simulink model "triplex_12B"  (R2024b)
settings: Solver=ode3  StartTime=0.0  StopTime=10.0  FixedStep=.1  RelTol=1e-3  EnableMultiTasking=on
settings Model: Creator=elliocm  LastModifiedBy=lukeubun
settings SolverCC: AlgebraicLoopSolver=TrustRegion
settings DataIOCC: LimitDataPoints=on  SaveFormat=StructureWithTime  SignalLoggingSaveFormat=ModelDataLogs  ReturnWorkspaceOutputs=off
settings OptimizationCC: ExpressionDepthLimit=2147483647  LifeSpan=inf
settings DebuggingCC: UnderspecifiedInitializationDetection=Classic  MergeDetectMultiDrivingBlocksExec=none  SolverPrmCheckMsg=warning  MultiTaskDSMMsg=warning  MultiTaskCondExecSysMsg=none  UnconnectedInputMsg=warning  UnconnectedOutputMsg=warning  UnconnectedLineMsg=warning  StateNameClashWarn=warning  SFUnexpectedBacktrackingDiag=warning  SFNoUnconditionalDefaultTransitionDiag=warning  SFExecutionAtInitializationDiag=none  ArithmeticOperatorsInVariantConditions=warning
settings HardwareCC: ProdBitPerPointer=32  ProdBitPerSizeT=32  ProdBitPerPtrDiffT=32  ProdLargestAtomicFloat=None  ProdIntDivRoundTo=Undefined  ProdEndianess=Unspecified  ProdWordSize=32  ProdHWDeviceType=32-bit Generic
settings ModelReferenceCC: PropagateSignalLabelsOutOfModel=off
settings SFSimCC: SimUseLocalCustomCode=off  CustomCodeUndefinedFunction=UseInterfaceOnly
settings RTWCC: RTWUseLocalCustomCode=off  GPUComputeCapability=3.5
settings CodeAppCC: StateflowObjectComments=on
settings GRTTargetCC: TargetLangStandard=C89/C90 (ANSI)
settings ConfigComp: CovMetricSettings=dw  CovSaveCumulativeToWorkspaceVar=on  CovSaveSingleToWorkspaceVar=on  CovExternalEMLEnable=off

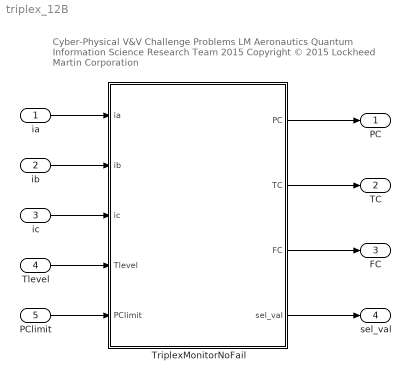
== system triplex_12B ==
  note: Cyber-Physical V&V Challenge Problems
      | LM Aeronautics Quantum Information Science Research Team 2015
      | Copyright © 2015 Lockheed Martin Corporation
  ia : Inport  OutDataTypeStr=double
  ib : Inport  Port=2  OutDataTypeStr=double
  ic : Inport  Port=3  OutDataTypeStr=double
  Tlevel : Inport  Port=4  OutDataTypeStr=double
  PClimit : Inport  Port=5  OutDataTypeStr=int32
  TriplexMonitorNoFail : Subsystem
  PC : Outport
  TC : Outport  Port=2
  FC : Outport  Port=3
  sel_val : Outport  Port=4
  wires:
  ia/1 -> TriplexMonitorNoFail/1(ia)
  ib/1 -> TriplexMonitorNoFail/2(ib)
  ic/1 -> TriplexMonitorNoFail/3(ic)
  Tlevel/1 -> TriplexMonitorNoFail/4(Tlevel)
  PClimit/1 -> TriplexMonitorNoFail/5(PClimit)
  TriplexMonitorNoFail/2(TC) -> TC/1
  TriplexMonitorNoFail/1(PC) -> PC/1
  TriplexMonitorNoFail/3(FC) -> FC/1
  TriplexMonitorNoFail/4(sel_val) -> sel_val/1

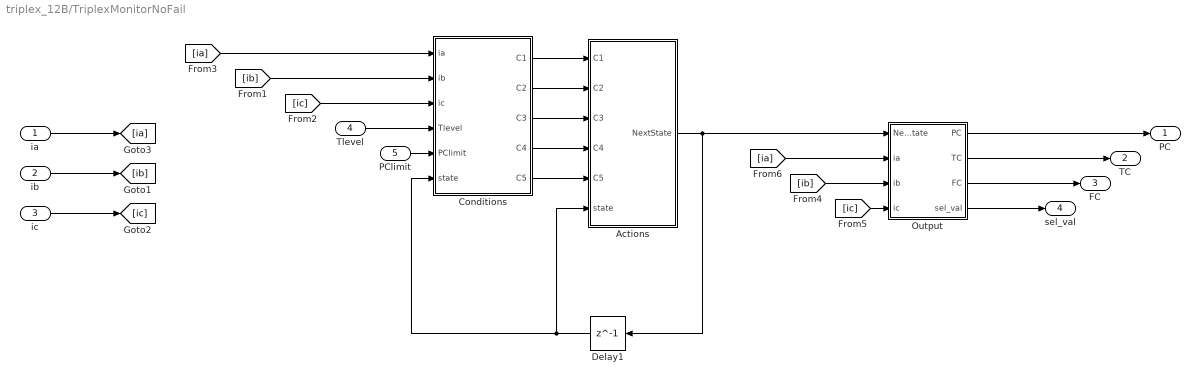
== system triplex_12B/TriplexMonitorNoFail ==
  ia : Inport
  ib : Inport  Port=2
  ic : Inport  Port=3
  Tlevel : Inport  Port=4
  PClimit : Inport  Port=5
  Actions : Subsystem
  Conditions : Subsystem
  Delay1 : Delay  DelayLength=1  InitialCondition=0
  Output : Subsystem
  PC : Outport
  TC : Outport  Port=2
  FC : Outport  Port=3
  sel_val : Outport  Port=4
  wires:
  Conditions/2(C2) -> Actions/2(C2)
  Conditions/5(C5) -> Actions/5(C5)
  Conditions/1(C1) -> Actions/1(C1)
  Conditions/4(C4) -> Actions/4(C4)
  Conditions/3(C3) -> Actions/3(C3)
  Tlevel/1 -> Conditions/4(Tlevel)
  PClimit/1 -> Conditions/5(PClimit)
  Output/2(TC) -> TC/1
  Output/1(PC) -> PC/1
  Output/3(FC) -> FC/1
  Actions/1(NextState) -> Delay1/1, Output/1(NextState)
  Delay1/1 -> Actions/6(state), Conditions/6(state)
  [ia] -> Conditions/1(ia)
  [ib] -> Conditions/2(ib)
  ib/1 -> [ib]
  ic/1 -> [ic]
  [ic] -> Conditions/3(ic)
  [ia] -> Output/2(ia)
  [ib] -> Output/3(ib)
  [ic] -> Output/4(ic)
  Output/4(sel_val) -> sel_val/1
  ia/1 -> [ia]

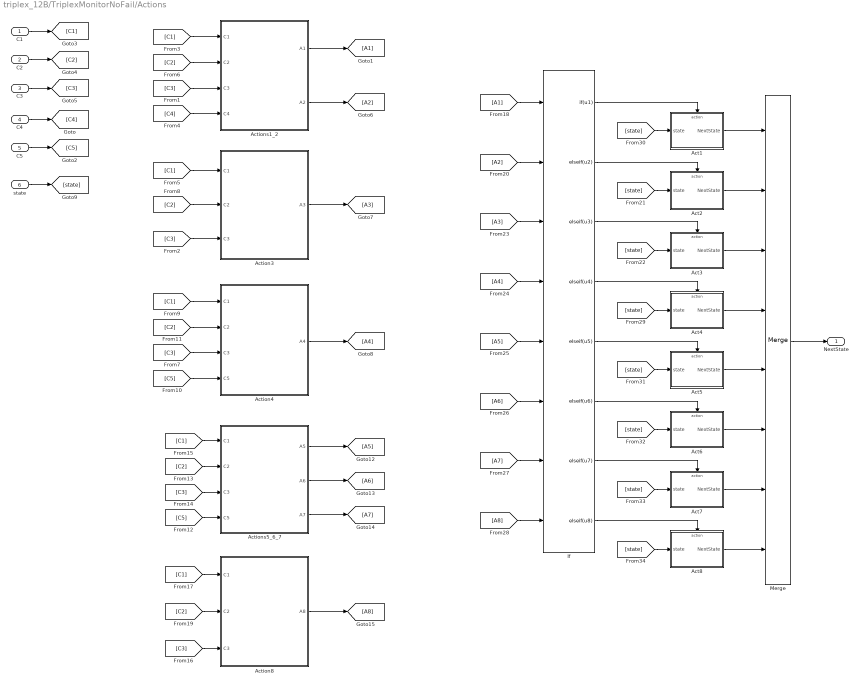
== system triplex_12B/TriplexMonitorNoFail/Actions ==
  C1 : Inport
  C2 : Inport  Port=2
  C3 : Inport  Port=3
  C4 : Inport  Port=4
  C5 : Inport  Port=5
  state : Inport  Port=6
  Act1 : Subsystem
  Act2 : Subsystem
  Act3 : Subsystem
  Act4 : Subsystem
  Act5 : Subsystem
  Act6 : Subsystem
  Act7 : Subsystem
  Act8 : Subsystem
  Action3 : Subsystem
  Action4 : Subsystem
  Action8 : Subsystem
  Actions1_2 : Subsystem
  Actions5_6_7 : Subsystem
  If : If  NumInputs=8  IfExpression=u1  ElseIfExpressions=u2, u3, u4, u5, u6, u7, u8  ShowElse=off
  Merge : Merge  Inputs=8
  NextState : Outport
  wires:
  C1/1 -> [C1]
  C5/1 -> [C5]
  C2/1 -> [C2]
  C3/1 -> [C3]
  C4/1 -> [C4]
  [C1] -> Actions1_2/1(C1)
  [C2] -> Actions1_2/2(C2)
  [C4] -> Actions1_2/4(C4)
  [C3] -> Actions1_2/3(C3)
  Actions1_2/2(A2) -> [A2]
  [C1] -> Action3/1(C1)
  [C2] -> Action3/2(C2)
  [C3] -> Action3/3(C3)
  Action4/1(A4) -> [A4]
  [C1] -> Action4/1(C1)
  [C2] -> Action4/2(C2)
  [C3] -> Action4/3(C3)
  [C5] -> Action4/4(C5)
  [C2] -> Actions5_6_7/2(C2)
  [C3] -> Actions5_6_7/3(C3)
  [C1] -> Actions5_6_7/1(C1)
  [C5] -> Actions5_6_7/4(C5)
  [C1] -> Action8/1(C1)
  [C2] -> Action8/2(C2)
  [C3] -> Action8/3(C3)
  Actions1_2/1(A1) -> [A1]
  Action3/1(A3) -> [A3]
  [A1] -> If/1
  If/1 -> Act1/Action
  [A2] -> If/2
  state/1 -> [state]
  If/2 -> Act2/Action
  If/3 -> Act3/Action
  [A3] -> If/3
  [A4] -> If/4
  [A5] -> If/5
  [A6] -> If/6
  [A7] -> If/7
  [A8] -> If/8
  If/4 -> Act4/Action
  Actions5_6_7/1(A5) -> [A5]
  Actions5_6_7/2(A6) -> [A6]
  Actions5_6_7/3(A7) -> [A7]
  Action8/1(A8) -> [A8]
  [state] -> Act1/1(state)
  If/5 -> Act5/Action
  If/6 -> Act6/Action
  If/7 -> Act7/Action
  If/8 -> Act8/Action
  Act1/1(NextState) -> Merge/1
  Act2/1(NextState) -> Merge/2
  Act3/1(NextState) -> Merge/3
  Act4/1(NextState) -> Merge/4
  Act5/1(NextState) -> Merge/5
  Act6/1(NextState) -> Merge/6
  Act7/1(NextState) -> Merge/7
  Act8/1(NextState) -> Merge/8
  Merge/1 -> NextState/1
  [state] -> Act2/1(state)
  [state] -> Act3/1(state)
  [state] -> Act4/1(state)
  [state] -> Act5/1(state)
  [state] -> Act6/1(state)
  [state] -> Act7/1(state)
  [state] -> Act8/1(state)

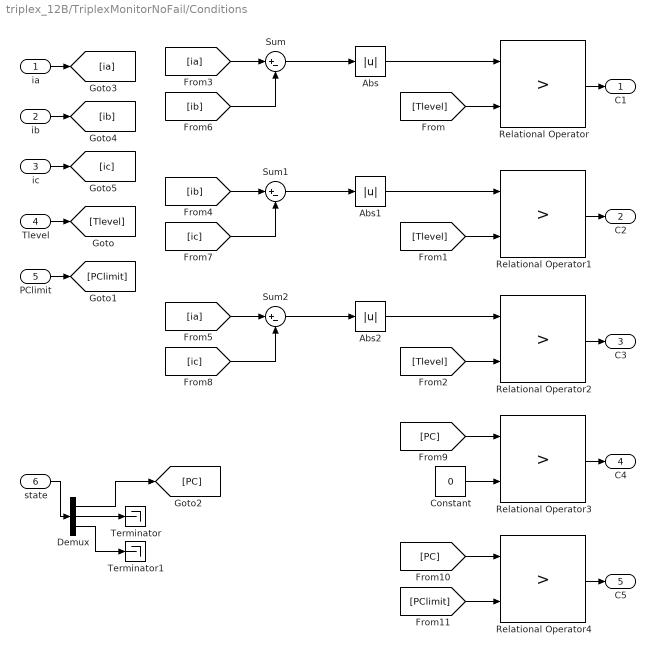
== system triplex_12B/TriplexMonitorNoFail/Conditions ==
  ia : Inport  Tag=ia
  ib : Inport  Port=2
  ic : Inport  Port=3
  Tlevel : Inport  Port=4
  PClimit : Inport  Port=5
  state : Inport  Port=6
  Abs : Abs  SaturateOnIntegerOverflow=off
  Abs1 : Abs  SaturateOnIntegerOverflow=off
  Abs2 : Abs  SaturateOnIntegerOverflow=off
  Constant : Constant  Value=0
  Demux : Demux  Outputs=3
  Relational Operator{,1..4} (5 alike) : RelationalOperator  Operator=>  OutDataTypeStr=boolean  InputSameDT=off
  Sum : Sum  Inputs=|+-
  Sum1 : Sum  Inputs=|+-
  Sum2 : Sum  Inputs=|+-
  Terminator : Terminator
  Terminator1 : Terminator
  C1 : Outport
  C2 : Outport  Port=2
  C3 : Outport  Port=3
  C4 : Outport  Port=4
  C5 : Outport  Port=5
  wires:
  Abs/1 -> Relational Operator/1
  Sum/1 -> Abs/1
  [Tlevel] -> Relational Operator/2
  Constant/1 -> Relational Operator3/2
  Abs1/1 -> Relational Operator1/1
  [Tlevel] -> Relational Operator1/2
  Sum1/1 -> Abs1/1
  Sum2/1 -> Abs2/1
  Abs2/1 -> Relational Operator2/1
  [Tlevel] -> Relational Operator2/2
  Relational Operator4/1 -> C5/1
  ib/1 -> [ib]
  [ia] -> Sum/1
  Relational Operator1/1 -> C2/1
  [PC] -> Relational Operator4/1
  Tlevel/1 -> [Tlevel]
  [ic] -> Sum1/2
  ia/1 -> [ia]
  ic/1 -> [ic]
  Relational Operator2/1 -> C3/1
  [ic] -> Sum2/2
  [ia] -> Sum2/1
  [ib] -> Sum/2
  [ib] -> Sum1/1
  [PC] -> Relational Operator3/1
  Relational Operator3/1 -> C4/1
  [PClimit] -> Relational Operator4/2
  PClimit/1 -> [PClimit]
  Relational Operator/1 -> C1/1
  state/1 -> Demux/1
  Demux/1 -> [PC]
  Demux/2 -> Terminator/1
  Demux/3 -> Terminator1/1

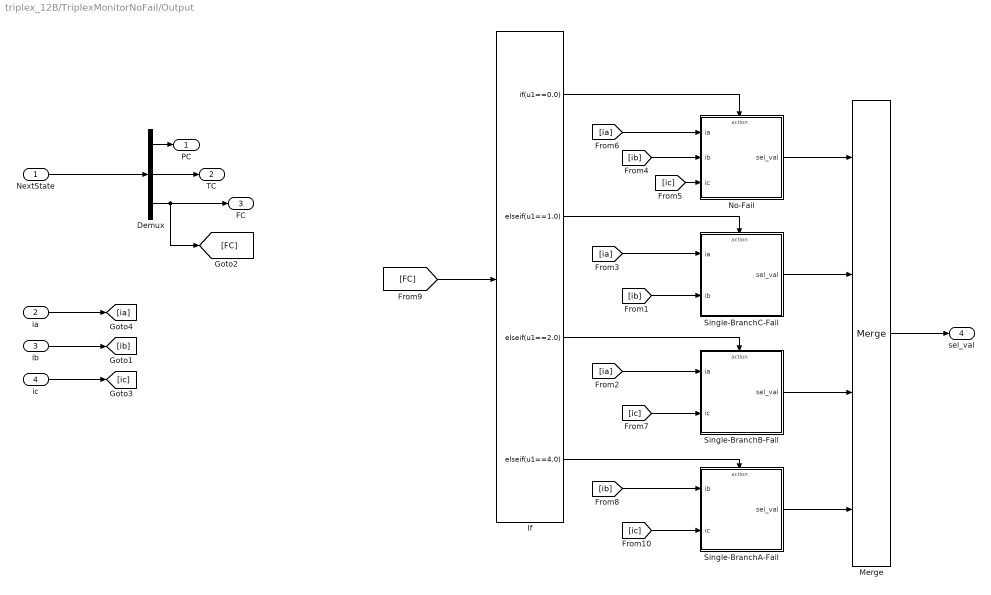
== system triplex_12B/TriplexMonitorNoFail/Output ==
  NextState : Inport
  ia : Inport  Port=2
  ib : Inport  Port=3
  ic : Inport  Port=4
  Demux : Demux  Outputs=3
  If : If  IfExpression=u1==0.0  ElseIfExpressions=u1==1.0, u1==2.0, u1==4.0  ShowElse=off
  Merge : Merge  Inputs=4
  No-Fail : Subsystem
  Single-BranchA-Fail : Subsystem
  Single-BranchB-Fail : Subsystem
  Single-BranchC-Fail : Subsystem
  PC : Outport
  TC : Outport  Port=2
  FC : Outport  Port=3
  sel_val : Outport  Port=4
  wires:
  NextState/1 -> Demux/1
  Demux/1 -> PC/1
  Demux/2 -> TC/1
  Demux/3 -> [FC], FC/1
  [FC] -> If/1
  If/1 -> No-Fail/Action
  ia/1 -> [ia]
  ib/1 -> [ib]
  ic/1 -> [ic]
  Merge/1 -> sel_val/1
  [ia] -> No-Fail/1(ia)
  [ib] -> No-Fail/2(ib)
  [ic] -> No-Fail/3(ic)
  If/2 -> Single-BranchC-Fail/Action
  [ia] -> Single-BranchC-Fail/1(ia)
  [ib] -> Single-BranchC-Fail/2(ib)
  If/3 -> Single-BranchB-Fail/Action
  [ia] -> Single-BranchB-Fail/1(ia)
  [ic] -> Single-BranchB-Fail/2(ic)
  If/4 -> Single-BranchA-Fail/Action
  [ib] -> Single-BranchA-Fail/1(ib)
  [ic] -> Single-BranchA-Fail/2(ic)
  No-Fail/1(sel_val) -> Merge/1
  Single-BranchC-Fail/1(sel_val) -> Merge/2
  Single-BranchB-Fail/1(sel_val) -> Merge/3
  Single-BranchA-Fail/1(sel_val) -> Merge/4

== system triplex_12B/TriplexMonitorNoFail/Actions/Act1 ==
  note: // Action 1: No pending failures
  state : Inport
  Action Port : ActionPort  ActionPortLabel=if(u1)
  Constant1 : Constant  Value=0  OutDataTypeStr=int32
  Demux : Demux  Outputs=3
  Mux : Mux  Inputs=3
  Signal Conversion : SignalConversion  OverrideOpt=off
  Terminator : Terminator
  NextState : Outport
  wires:
  state/1 -> [state]
  Signal Conversion/1 -> NextState/1
  Mux/1 -> Signal Conversion/1
  [state] -> Demux/1
  Demux/2 -> Mux/2
  Demux/3 -> Mux/3
  Constant1/1 -> Mux/1
  Demux/1 -> Terminator/1

== system triplex_12B/TriplexMonitorNoFail/Actions/Act2 ==
  note: // Action 2: Failure pending but no miscompares
  state : Inport
  Action Port : ActionPort  ActionPortLabel=elseif(u2)
  Constant1 : Constant  OutDataTypeStr=int32
  Demux : Demux  Outputs=3
  Mux : Mux  Inputs=3
  Signal Conversion : SignalConversion  OverrideOpt=off
  Sum : Sum  Inputs=-+|
  NextState : Outport
  wires:
  state/1 -> [state]
  Constant1/1 -> Sum/1
  Signal Conversion/1 -> NextState/1
  Mux/1 -> Signal Conversion/1
  [state] -> Demux/1
  Demux/2 -> Mux/2
  Demux/3 -> Mux/3
  Sum/1 -> Mux/1
  Demux/1 -> Sum/2

== system triplex_12B/TriplexMonitorNoFail/Actions/Act3 ==
  note: // Action 3: Do nothing there is only 1 miscompare
  state : Inport
  Action Port : ActionPort  ActionPortLabel=elseif( u3)
  NextState : Outport
  wires:
  state/1 -> NextState/1

== system triplex_12B/TriplexMonitorNoFail/Actions/Act4 ==
  note: // Action 4: Failure pending
  state : Inport
  Action Port : ActionPort  ActionPortLabel=elseif( u4)
  Constant1 : Constant  OutDataTypeStr=int32
  Demux : Demux  Outputs=3
  Mux : Mux  Inputs=3
  Signal Conversion : SignalConversion  OverrideOpt=off
  Sum : Sum  Inputs=++|
  Sum1 : Sum  Inputs=|++
  NextState : Outport
  wires:
  state/1 -> [state]
  Signal Conversion/1 -> NextState/1
  Mux/1 -> Signal Conversion/1
  [state] -> Demux/1
  Demux/2 -> Sum/2
  Constant1/1 -> Sum1/2, Sum/1
  Demux/1 -> Sum1/1
  Sum1/1 -> Mux/1
  Sum/1 -> Mux/2
  Demux/3 -> Mux/3

== system triplex_12B/TriplexMonitorNoFail/Actions/Act5 ==
  note: // Action 5: Failure latched (branch B)
  state : Inport
  Action Port : ActionPort  ActionPortLabel=elseif( u5)
  Constant : Constant  Value=0  OutDataTypeStr=int32
  Constant1 : Constant  Value=2  OutDataTypeStr=int32
  Mux : Mux  Inputs=3
  Selector : Selector  InputPortWidth=3  IndexOptions=Index vector (dialog)  Indices=[2]  OutputSizes=1
  Signal Conversion : SignalConversion  OverrideOpt=off
  NextState : Outport
  wires:
  state/1 -> [state]
  Mux/1 -> Signal Conversion/1
  Constant/1 -> Mux/1
  Constant1/1 -> Mux/3
  Selector/1 -> Mux/2
  [state] -> Selector/1
  Signal Conversion/1 -> NextState/1

== system triplex_12B/TriplexMonitorNoFail/Actions/Act6 ==
  note: // Action 6: Failure latched (branch A)
  state : Inport
  Action Port : ActionPort  ActionPortLabel=elseif( u6)
  Constant : Constant  Value=0  OutDataTypeStr=int32
  Constant1 : Constant  Value=4  OutDataTypeStr=int32
  Mux : Mux  Inputs=3
  Selector : Selector  InputPortWidth=3  IndexOptions=Index vector (dialog)  Indices=[2]  OutputSizes=1
  Signal Conversion : SignalConversion  OverrideOpt=off
  NextState : Outport
  wires:
  state/1 -> [state]
  Mux/1 -> Signal Conversion/1
  Constant/1 -> Mux/1
  Constant1/1 -> Mux/3
  Selector/1 -> Mux/2
  [state] -> Selector/1
  Signal Conversion/1 -> NextState/1

== system triplex_12B/TriplexMonitorNoFail/Actions/Act7 ==
  note: /// Action 7: Failure latched (branch C)
  state : Inport
  Action Port : ActionPort  ActionPortLabel=elseif( u7)
  Constant : Constant  Value=0  OutDataTypeStr=int32
  Constant1 : Constant  OutDataTypeStr=int32
  Mux : Mux  Inputs=3
  Selector : Selector  InputPortWidth=3  IndexOptions=Index vector (dialog)  Indices=[2]  OutputSizes=1
  Signal Conversion : SignalConversion  OverrideOpt=off
  NextState : Outport
  wires:
  state/1 -> [state]
  Mux/1 -> Signal Conversion/1
  Constant/1 -> Mux/1
  Constant1/1 -> Mux/3
  Selector/1 -> Mux/2
  [state] -> Selector/1
  Signal Conversion/1 -> NextState/1

== system triplex_12B/TriplexMonitorNoFail/Actions/Act8 ==
  note: // Action 8: All branches miscompare
  state : Inport
  Action Port : ActionPort  ActionPortLabel=elseif( u8)
  Constant1 : Constant  OutDataTypeStr=int32
  Demux : Demux  Outputs=3
  Mux : Mux  Inputs=3
  Signal Conversion : SignalConversion  OverrideOpt=off
  Sum1 : Sum  Inputs=++|
  NextState : Outport
  wires:
  state/1 -> [state]
  Mux/1 -> Signal Conversion/1
  Demux/1 -> Mux/1
  Demux/3 -> Mux/3
  Sum1/1 -> Mux/2
  Constant1/1 -> Sum1/1
  Demux/2 -> Sum1/2
  Signal Conversion/1 -> NextState/1
  [state] -> Demux/1

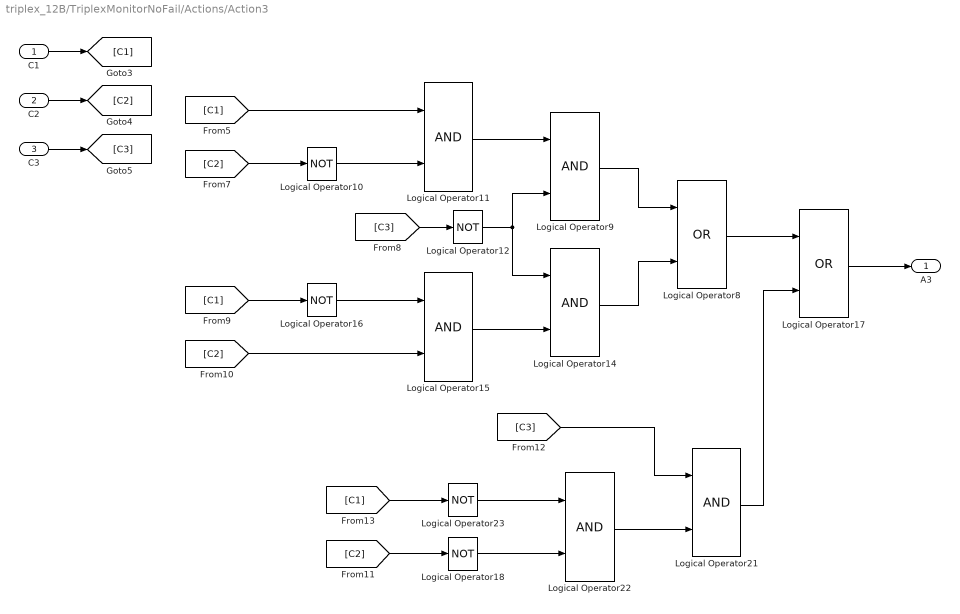
== system triplex_12B/TriplexMonitorNoFail/Actions/Action3 ==
  C1 : Inport
  C2 : Inport  Port=2
  C3 : Inport  Port=3
  Logical Operator{10,12,16,18,23} (5 alike) : Logic  Operator=NOT  Inputs=1  AllPortsSameDT=off  OutDataTypeStr=boolean
  Logical Operator{9,11,14..15,21..22} (6 alike) : Logic  AllPortsSameDT=off  OutDataTypeStr=boolean
  Logical Operator17 : Logic  Operator=OR  AllPortsSameDT=off  OutDataTypeStr=boolean
  Logical Operator8 : Logic  Operator=OR  AllPortsSameDT=off  OutDataTypeStr=boolean
  A3 : Outport
  wires:
  [C1] -> Logical Operator11/1
  [C2] -> Logical Operator10/1
  Logical Operator10/1 -> Logical Operator11/2
  Logical Operator12/1 -> Logical Operator9/2, Logical Operator14/1
  [C3] -> Logical Operator12/1
  Logical Operator11/1 -> Logical Operator9/1
  Logical Operator16/1 -> Logical Operator15/1
  [C1] -> Logical Operator16/1
  Logical Operator9/1 -> Logical Operator8/1
  [C2] -> Logical Operator15/2
  Logical Operator15/1 -> Logical Operator14/2
  Logical Operator14/1 -> Logical Operator8/2
  Logical Operator8/1 -> Logical Operator17/1
  Logical Operator21/1 -> Logical Operator17/2
  [C2] -> Logical Operator18/1
  [C1] -> Logical Operator23/1
  [C3] -> Logical Operator21/1
  Logical Operator23/1 -> Logical Operator22/1
  Logical Operator22/1 -> Logical Operator21/2
  Logical Operator18/1 -> Logical Operator22/2
  Logical Operator17/1 -> A3/1
  C1/1 -> [C1]
  C2/1 -> [C2]
  C3/1 -> [C3]

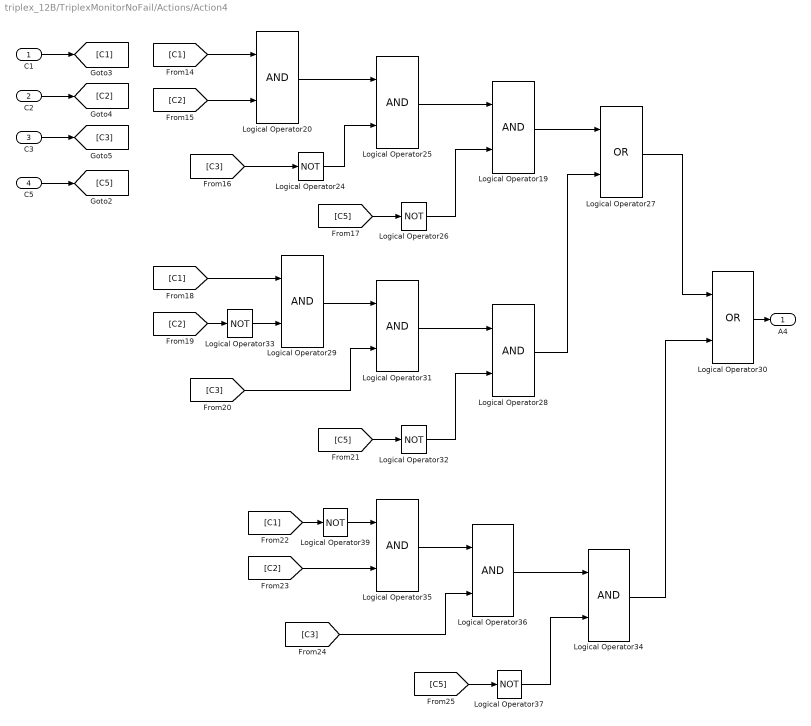
== system triplex_12B/TriplexMonitorNoFail/Actions/Action4 ==
  C1 : Inport
  C2 : Inport  Port=2
  C3 : Inport  Port=3
  C5 : Inport  Port=4
  Logical Operator{19..20,25,28..29,31,34..36} (9 alike) : Logic  AllPortsSameDT=off  OutDataTypeStr=boolean
  Logical Operator{24,26,32..33,37,39} (6 alike) : Logic  Operator=NOT  Inputs=1  AllPortsSameDT=off  OutDataTypeStr=boolean
  Logical Operator27 : Logic  Operator=OR  AllPortsSameDT=off  OutDataTypeStr=boolean
  Logical Operator30 : Logic  Operator=OR  AllPortsSameDT=off  OutDataTypeStr=boolean
  A4 : Outport
  wires:
  [C3] -> Logical Operator31/2
  Logical Operator31/1 -> Logical Operator28/1
  [C5] -> Logical Operator32/1
  Logical Operator32/1 -> Logical Operator28/2
  [C1] -> Logical Operator29/1
  Logical Operator28/1 -> Logical Operator27/2
  Logical Operator29/1 -> Logical Operator31/1
  [C2] -> Logical Operator33/1
  [C3] -> Logical Operator24/1
  [C2] -> Logical Operator20/2
  [C1] -> Logical Operator20/1
  Logical Operator20/1 -> Logical Operator25/1
  Logical Operator30/1 -> A4/1
  Logical Operator26/1 -> Logical Operator19/2
  Logical Operator33/1 -> Logical Operator29/2
  Logical Operator25/1 -> Logical Operator19/1
  [C5] -> Logical Operator26/1
  Logical Operator19/1 -> Logical Operator27/1
  Logical Operator24/1 -> Logical Operator25/2
  Logical Operator36/1 -> Logical Operator34/1
  Logical Operator27/1 -> Logical Operator30/1
  Logical Operator37/1 -> Logical Operator34/2
  [C5] -> Logical Operator37/1
  [C3] -> Logical Operator36/2
  Logical Operator39/1 -> Logical Operator35/1
  Logical Operator35/1 -> Logical Operator36/1
  [C1] -> Logical Operator39/1
  Logical Operator34/1 -> Logical Operator30/2
  [C2] -> Logical Operator35/2
  C1/1 -> [C1]
  C5/1 -> [C5]
  C2/1 -> [C2]
  C3/1 -> [C3]

== system triplex_12B/TriplexMonitorNoFail/Actions/Action8 ==
  C1 : Inport
  C2 : Inport  Port=2
  C3 : Inport  Port=3
  Logical Operator3 : Logic  AllPortsSameDT=off  OutDataTypeStr=boolean
  Logical Operator4 : Logic  AllPortsSameDT=off  OutDataTypeStr=boolean
  A8 : Outport
  wires:
  Logical Operator3/1 -> Logical Operator4/1
  C3/1 -> Logical Operator4/2
  C1/1 -> Logical Operator3/1
  C2/1 -> Logical Operator3/2
  Logical Operator4/1 -> A8/1

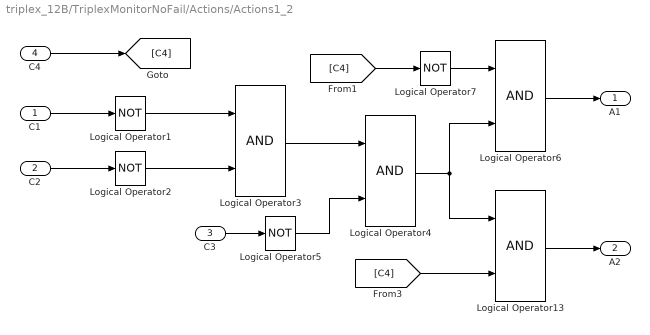
== system triplex_12B/TriplexMonitorNoFail/Actions/Actions1_2 ==
  C1 : Inport
  C2 : Inport  Port=2
  C3 : Inport  Port=3
  C4 : Inport  Port=4
  Logical Operator{1..2,5,7} (4 alike) : Logic  Operator=NOT  Inputs=1  AllPortsSameDT=off  OutDataTypeStr=boolean
  Logical Operator{3..4,6,13} (4 alike) : Logic  AllPortsSameDT=off  OutDataTypeStr=boolean
  A1 : Outport
  A2 : Outport  Port=2
  wires:
  C2/1 -> Logical Operator2/1
  Logical Operator4/1 -> Logical Operator6/2, Logical Operator13/1
  Logical Operator2/1 -> Logical Operator3/2
  [C4] -> Logical Operator13/2
  C1/1 -> Logical Operator1/1
  Logical Operator1/1 -> Logical Operator3/1
  Logical Operator6/1 -> A1/1
  Logical Operator7/1 -> Logical Operator6/1
  Logical Operator3/1 -> Logical Operator4/1
  [C4] -> Logical Operator7/1
  Logical Operator13/1 -> A2/1
  Logical Operator5/1 -> Logical Operator4/2
  C3/1 -> Logical Operator5/1
  C4/1 -> [C4]

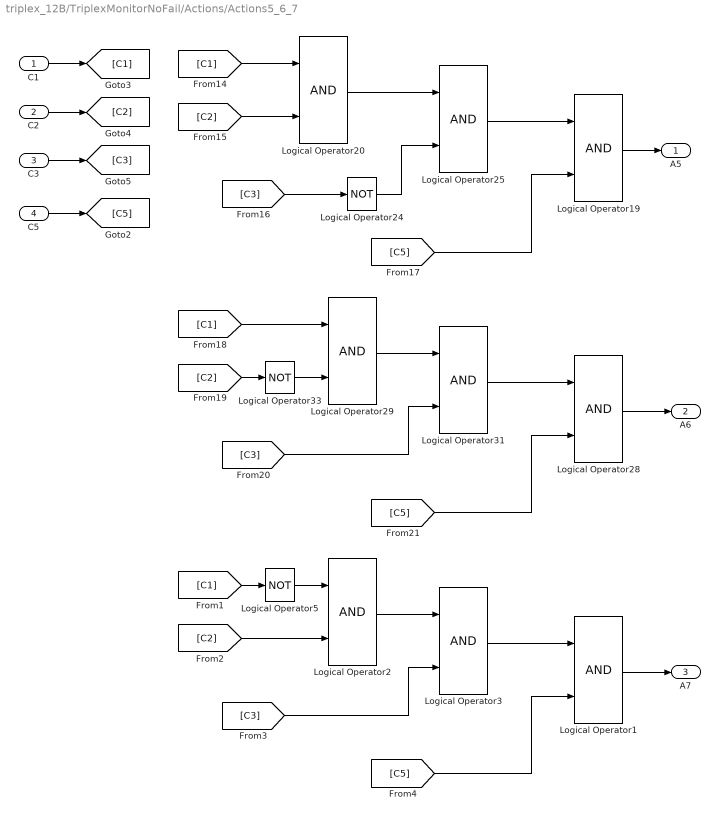
== system triplex_12B/TriplexMonitorNoFail/Actions/Actions5_6_7 ==
  C1 : Inport
  C2 : Inport  Port=2
  C3 : Inport  Port=3
  C5 : Inport  Port=4
  Logical Operator{1..3,19..20,25,28..29,31} (9 alike) : Logic  AllPortsSameDT=off  OutDataTypeStr=boolean
  Logical Operator24 : Logic  Operator=NOT  Inputs=1  AllPortsSameDT=off  OutDataTypeStr=boolean
  Logical Operator33 : Logic  Operator=NOT  Inputs=1  AllPortsSameDT=off  OutDataTypeStr=boolean
  Logical Operator5 : Logic  Operator=NOT  Inputs=1  AllPortsSameDT=off  OutDataTypeStr=boolean
  A5 : Outport
  A6 : Outport  Port=2
  A7 : Outport  Port=3
  wires:
  [C3] -> Logical Operator31/2
  Logical Operator31/1 -> Logical Operator28/1
  [C5] -> Logical Operator28/2
  [C1] -> Logical Operator29/1
  Logical Operator29/1 -> Logical Operator31/1
  [C2] -> Logical Operator33/1
  [C3] -> Logical Operator24/1
  [C2] -> Logical Operator20/2
  [C1] -> Logical Operator20/1
  Logical Operator20/1 -> Logical Operator25/1
  [C5] -> Logical Operator19/2
  Logical Operator33/1 -> Logical Operator29/2
  Logical Operator25/1 -> Logical Operator19/1
  Logical Operator24/1 -> Logical Operator25/2
  C1/1 -> [C1]
  C5/1 -> [C5]
  C2/1 -> [C2]
  C3/1 -> [C3]
  Logical Operator19/1 -> A5/1
  Logical Operator28/1 -> A6/1
  [C3] -> Logical Operator3/2
  Logical Operator3/1 -> Logical Operator1/1
  [C5] -> Logical Operator1/2
  [C1] -> Logical Operator5/1
  Logical Operator2/1 -> Logical Operator3/1
  [C2] -> Logical Operator2/2
  Logical Operator1/1 -> A7/1
  Logical Operator5/1 -> Logical Operator2/1

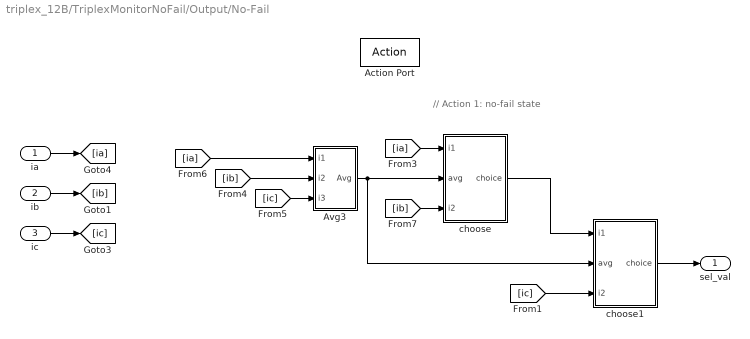
== system triplex_12B/TriplexMonitorNoFail/Output/No-Fail ==
  note: // Action 1: no-fail state
  ia : Inport
  ib : Inport  Port=2
  ic : Inport  Port=3
  Action Port : ActionPort  ActionPortLabel=if(u1==0.0)
  Avg3 : Subsystem
  choose : Subsystem
  choose1 : Subsystem
  sel_val : Outport
  wires:
  ia/1 -> [ia]
  ib/1 -> [ib]
  ic/1 -> [ic]
  [ia] -> Avg3/1(i1)
  [ib] -> Avg3/2(i2)
  [ic] -> Avg3/3(i3)
  [ia] -> choose/1(i1)
  Avg3/1(Avg) -> choose1/2(avg), choose/2(avg)
  [ib] -> choose/3(i2)
  choose/1(choice) -> choose1/1(i1)
  [ic] -> choose1/3(i2)
  choose1/1(choice) -> sel_val/1

== system triplex_12B/TriplexMonitorNoFail/Output/Single-BranchA-Fail ==
  note: // Action 4: Single-BranchA-Fail
  ib : Inport
  ic : Inport  Port=2
  Action Port : ActionPort  ActionPortLabel=elseif( u1==4.0)
  Avg2 : Subsystem
  sel_val : Outport
  wires:
  Avg2/1(Avg) -> sel_val/1
  [ic] -> Avg2/2(i2)
  [ib] -> Avg2/1(i1)
  ic/1 -> [ic]
  ib/1 -> [ib]

== system triplex_12B/TriplexMonitorNoFail/Output/Single-BranchB-Fail ==
  note: // Action 3: Single-BranchB-Fail
  ia : Inport
  ic : Inport  Port=2
  Action Port : ActionPort  ActionPortLabel=elseif( u1==2.0)
  Avg2 : Subsystem
  sel_val : Outport
  wires:
  ia/1 -> [ia]
  ic/1 -> [ic]
  [ia] -> Avg2/1(i1)
  [ic] -> Avg2/2(i2)
  Avg2/1(Avg) -> sel_val/1

== system triplex_12B/TriplexMonitorNoFail/Output/Single-BranchC-Fail ==
  note: // Action 2: Single-BranchC-Fail
  ia : Inport
  ib : Inport  Port=2
  Action Port : ActionPort  ActionPortLabel=elseif(u1==1.0)
  Avg2 : Subsystem
  sel_val : Outport
  wires:
  Avg2/1(Avg) -> sel_val/1
  [ib] -> Avg2/2(i2)
  [ia] -> Avg2/1(i1)
  ib/1 -> [ib]
  ia/1 -> [ia]

== system triplex_12B/TriplexMonitorNoFail/Output/No-Fail/Avg3 ==
  i1 : Inport
  i2 : Inport  Port=2
  i3 : Inport  Port=3
  Constant : Constant  Value=3.0
  Divide : Product  Inputs=*/
  Sum : Sum  Inputs=|++
  Sum1 : Sum  Inputs=|++
  Avg : Outport
  wires:
  Sum1/1 -> Divide/1
  Constant/1 -> Divide/2
  i2/1 -> Sum/2
  Sum/1 -> Sum1/1
  Divide/1 -> Avg/1
  i3/1 -> Sum1/2
  i1/1 -> Sum/1

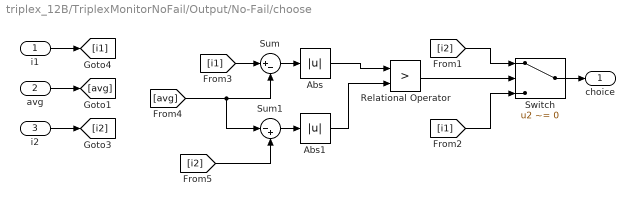
== system triplex_12B/TriplexMonitorNoFail/Output/No-Fail/choose ==
  i1 : Inport
  avg : Inport  Port=2
  i2 : Inport  Port=3
  Abs : Abs  SaturateOnIntegerOverflow=off
  Abs1 : Abs  SaturateOnIntegerOverflow=off
  Relational Operator : RelationalOperator  Operator=>  OutDataTypeStr=boolean  InputSameDT=off
  Sum : Sum  Inputs=|+-
  Sum1 : Sum  Inputs=|-+
  Switch : Switch  Criteria=u2 ~= 0  SaturateOnIntegerOverflow=off  InputSameDT=off
  choice : Outport
  wires:
  Abs/1 -> Relational Operator/1
  Switch/1 -> choice/1
  [i1] -> Sum/1
  [i1] -> Switch/3
  [i2] -> Switch/1
  Abs1/1 -> Relational Operator/2
  Sum1/1 -> Abs1/1
  Relational Operator/1 -> Switch/2
  [i2] -> Sum1/2
  Sum/1 -> Abs/1
  [avg] -> Sum1/1, Sum/2
  i1/1 -> [i1]
  avg/1 -> [avg]
  i2/1 -> [i2]

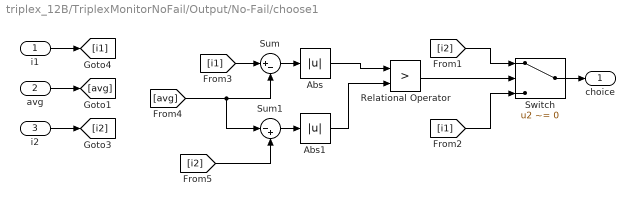
== system triplex_12B/TriplexMonitorNoFail/Output/No-Fail/choose1 ==
  i1 : Inport
  avg : Inport  Port=2
  i2 : Inport  Port=3
  Abs : Abs  SaturateOnIntegerOverflow=off
  Abs1 : Abs  SaturateOnIntegerOverflow=off
  Relational Operator : RelationalOperator  Operator=>  OutDataTypeStr=boolean  InputSameDT=off
  Sum : Sum  Inputs=|+-
  Sum1 : Sum  Inputs=|-+
  Switch : Switch  Criteria=u2 ~= 0  SaturateOnIntegerOverflow=off  InputSameDT=off
  choice : Outport
  wires:
  i2/1 -> [i2]
  avg/1 -> [avg]
  i1/1 -> [i1]
  [avg] -> Sum/2, Sum1/1
  Sum/1 -> Abs/1
  [i2] -> Sum1/2
  Relational Operator/1 -> Switch/2
  Sum1/1 -> Abs1/1
  Abs1/1 -> Relational Operator/2
  [i2] -> Switch/1
  [i1] -> Switch/3
  [i1] -> Sum/1
  Switch/1 -> choice/1
  Abs/1 -> Relational Operator/1

== system triplex_12B/TriplexMonitorNoFail/Output/Single-BranchA-Fail/Avg2 ==
  i1 : Inport
  i2 : Inport  Port=2
  Constant : Constant  Value=2.0
  Divide : Product  Inputs=*/
  Sum : Sum  Inputs=|++
  Avg : Outport
  wires:
  i1/1 -> Sum/1
  Divide/1 -> Avg/1
  i2/1 -> Sum/2
  Constant/1 -> Divide/2
  Sum/1 -> Divide/1

== system triplex_12B/TriplexMonitorNoFail/Output/Single-BranchB-Fail/Avg2 ==
  i1 : Inport
  i2 : Inport  Port=2
  Constant : Constant  Value=2.0
  Divide : Product  Inputs=*/
  Sum : Sum  Inputs=|++
  Avg : Outport
  wires:
  Sum/1 -> Divide/1
  Constant/1 -> Divide/2
  i2/1 -> Sum/2
  Divide/1 -> Avg/1
  i1/1 -> Sum/1

== system triplex_12B/TriplexMonitorNoFail/Output/Single-BranchC-Fail/Avg2 ==
  i1 : Inport
  i2 : Inport  Port=2
  Constant : Constant  Value=2.0
  Divide : Product  Inputs=*/
  Sum : Sum  Inputs=|++
  Avg : Outport
  wires:
  i1/1 -> Sum/1
  Divide/1 -> Avg/1
  i2/1 -> Sum/2
  Constant/1 -> Divide/2
  Sum/1 -> Divide/1
